simulink model "ECE556Lab1Task5"  (R2013b)
settings: Solver=ode45  StartTime=0.0  StopTime=5  MaxStep=.01  RelTol=1e-3
libraries: simulink x1
settings Model: Creator=Ben  LastModifiedBy=Ben

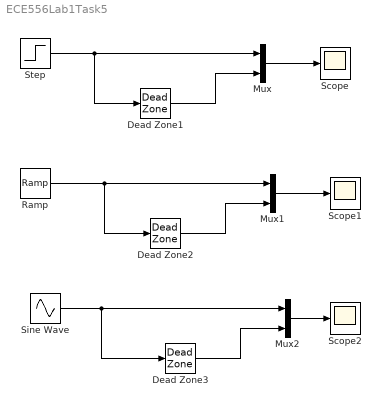
== system ECE556Lab1Task5 ==
  Dead Zone1 : DeadZone  LowerValue=-1.5  UpperValue=1.5  SaturateOnIntegerOverflow=on
  Dead Zone2 : DeadZone  LowerValue=-1.5  UpperValue=1.5  SaturateOnIntegerOverflow=on
  Dead Zone3 : DeadZone  LowerValue=-1.5  UpperValue=1.5  SaturateOnIntegerOverflow=on
  Mux : Mux  Inputs=2
  Mux1 : Mux  Inputs=2
  Mux2 : Mux  Inputs=2
  Ramp : simulink/Sources/Ramp  slope=1  start=0  X0=0
  Scope : Scope
  Scope1 : Scope
  Scope2 : Scope
      settings: SaveName=ScopeData2
  Sine Wave : Sin  Amplitude=5  Frequency=2*pi  SampleTime=0
  Step : Step  After=5  SampleTime=0
  wires:
  Mux/1 -> Scope/1
  Step/1 -> Dead Zone1/1, Mux/1
  Dead Zone1/1 -> Mux/2
  Mux1/1 -> Scope1/1
  Dead Zone2/1 -> Mux1/2
  Ramp/1 -> Dead Zone2/1, Mux1/1
  Mux2/1 -> Scope2/1
  Dead Zone3/1 -> Mux2/2
  Sine Wave/1 -> Mux2/1, Dead Zone3/1
